simulink model "Megaphone_And_Car_Sim"  (R2025b)
settings: Solver=VariableStepAuto  StartTime=0.0  StopTime=20  MaxStep=0.01  RelTol=1e-3
libraries: simulink x1
settings Model: Creator=night  LastModifiedBy=night

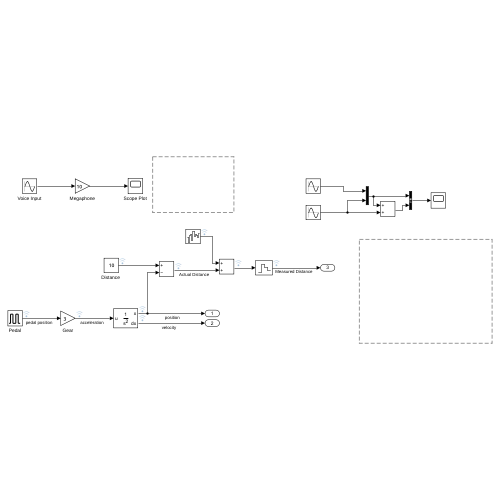
[thumbnail: Simulink's stored preview of the top-level diagram]
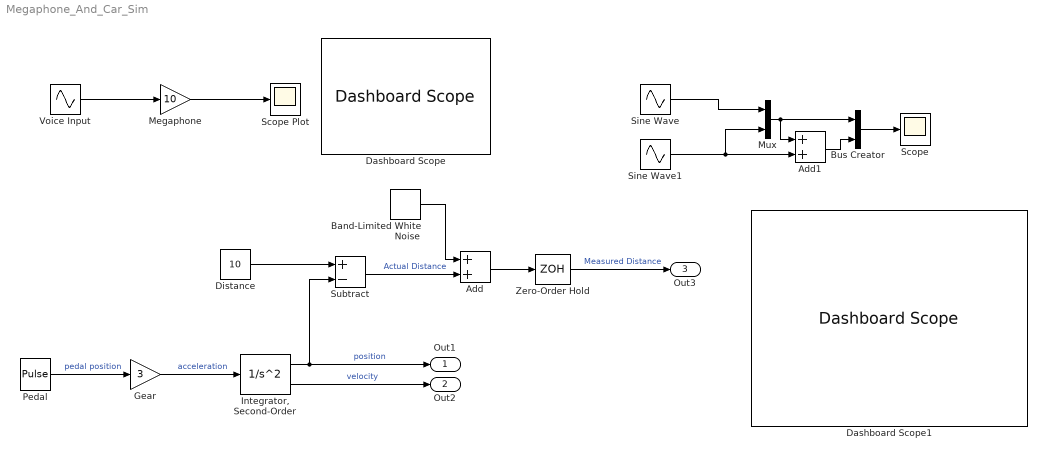
== system Megaphone_And_Car_Sim ==
  Add : Sum
  Add1 : Sum
  Band-Limited White Noise : simulink/Sources/Band-Limited White Noise  Cov=[0.1]  Ts=0.1  seed=[23341]
  Bus Creator : BusCreator  Inputs=2
  Dashboard Scope : DashboardScope  FontColor=[0.0, 0.0, 0.0]
  Dashboard Scope1 : DashboardScope  FontColor=[0.0, 0.0, 0.0]
  "Distance " : Constant  Value=10
  Gear : Gain  Gain=3
  "Integrator, Second-Order" : SecondOrderIntegrator
  Megaphone : Gain  Gain=10
  Mux : Mux  Inputs=2
  Pedal : DiscretePulseGenerator  PulseType=Time based  Period=10  PulseWidth=5
  Scope : Scope
      settings: ActiveDisplayYMinimum=-4.9999963796046618  ActiveDisplayYMaximum=4.9999981885420057
  Scope Plot : Scope
  Sine Wave : Sin  SampleTime=0
  Sine Wave1 : Sin  Amplitude=2  SampleTime=0
  Subtract : Sum  Inputs=+-
  Voice Input : Sin  SampleTime=0
  Zero-Order Hold : ZeroOrderHold  SampleTime=-1
  Out1 : Outport
  Out2 : Outport  Port=2
  Out3 : Outport  Port=3
  wires:
  Voice Input/1 -> Megaphone/1
  Megaphone/1 -> Scope Plot/1
  "Integrator, Second-Order"/1 -> Subtract/2, Out1/1  "position"
  "Integrator, Second-Order"/2 -> Out2/1  "velocity"
  Gear/1 -> "Integrator, Second-Order"/1  "acceleration"
  Pedal/1 -> Gear/1  "pedal position"
  "Distance "/1 -> Subtract/1
  Subtract/1 -> Add/2  "Actual Distance"
  Band-Limited White Noise/1 -> Add/1
  Add/1 -> Zero-Order Hold/1
  Zero-Order Hold/1 -> Out3/1  "Measured Distance"
  Sine Wave/1 -> Mux/1
  Sine Wave1/1 -> Add1/2, Mux/2
  Mux/1 -> Add1/1, Bus Creator/1
  Bus Creator/1 -> Scope/1
  Add1/1 -> Bus Creator/2
